simulink model "dummy"  (R2024b)
settings: Solver=VariableStepAuto  StartTime=0.0  StopTime=total_time  MaxStep=0.001  RelTol=1e-3
values from neighbouring files (symbols this model uses):
  D = diag([0.001, 0.001, 0.0175/6, 0.0175/6, 0.0175/6, 0.0175/6*Ts, 0.0175/6*Ts].^2)    [EX_opt_2.m]
  d = d_nom    (= 0.165)    [EX_opt_2.m]
  omega_wheels = sim_Tc_18.measures.signals.values(:,4:5)    [EX_opt_2.m]
  P_INIT_EKF = diag([0.001, 0.001, 0.0175/6, 0.0175/6, 0.0175/6, 0.0175/6*Ts, 0.0175/6*Ts].^2)    [EX_opt_2.m]
  PHI_INIT = [0; 0]    [EX_opt_2.m]
  prob_gps_loss = 0    [EX_opt_2.m]
  q = sim_Tc_18.measures.signals.values(:,1:3)    [EX_opt_2.m]
  Q_INIT_LOC = Q_INIT    [EX_opt_2.m]
  r = r_nom    (= 0.03)    [EX_opt_2.m]
  R_2 = diag([ENCODER_QUANTIZATION/6,ENCODER_QUANTIZATION/6].^2)    [EX_opt_2.m]
  R_5 = diag(([0.001, 0.001, 0.001, ENCODER_QUANTIZATION/6,ENCODER_QUANTIZATION/6]).^2)    [EX_opt_2.m]
  T_s = 0.04    [EX_opt_2.m]
  Ta = 1    [EX_opt_2.m]
  Tc = 18    [EX_opt_2.m]
  Ts = 0.04    [EX_opt_2.m]
  Z_INIT_EKF = [0; 0; 0; 0; 0; 0; 0]    [EX_opt_2.m]
undefined symbols (not defined in the file or in its folder): t_law
settings Model: Creator=alberto  LastModifiedBy=Enrico
settings DataIOCC: ReturnWorkspaceOutputs=off
settings RTWCC: GPUComputeCapability=3.5

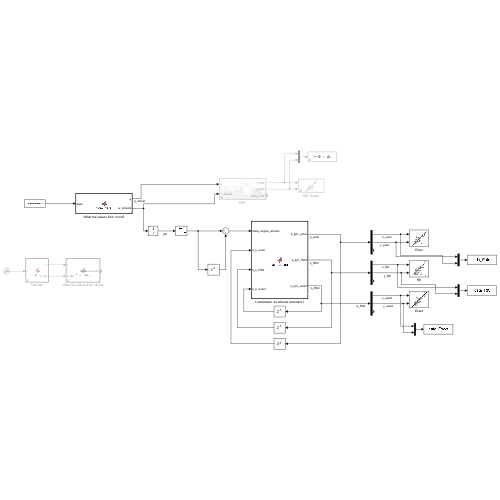
[thumbnail: Simulink's stored preview of the top-level diagram]
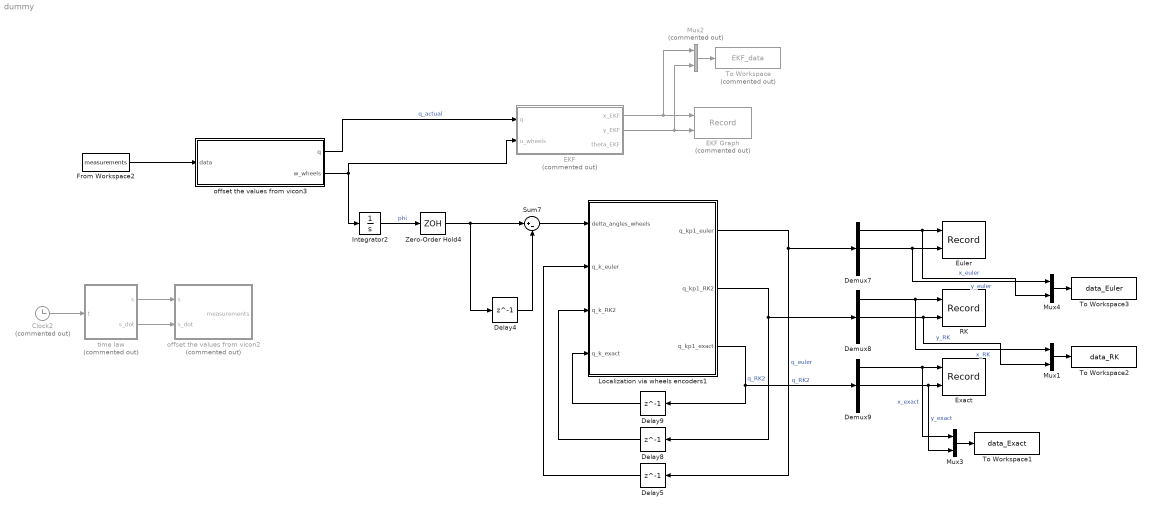
== system dummy ==
  Clock2 : Clock  Commented=on
      settings: Decimation=1/T_s
  Delay4 : Delay  DelayLength=1  InitialCondition=[0;0]  SampleTime=T_s
  Delay5 : Delay  DelayLength=1  InitialCondition=Q_INIT_LOC
  Delay8 : Delay  DelayLength=1  InitialCondition=Q_INIT_LOC
  Delay9 : Delay  DelayLength=1  InitialCondition=Q_INIT_LOC
  Demux7 : Demux  Outputs=3
  Demux8 : Demux  Outputs=3
  Demux9 : Demux  Outputs=3
  EKF : Subsystem  Commented=on
  EKF Graph : Record  Commented=on  FileSettingsInternal="{\"entries\":[{\"content\":{\"excelSettings\":{\"content\":{},\"type\":\"Streamout.ExcelSettings\"}},\"type\":\"Streamout.FileSettingStorage\",\"uuid\":\"\"}],\"packageUris\":[\"http:\\/\\/schema.mathworks.com\\/mf0\\/streamout_blocks\\/R2020a\"],\"version\":\"1.0\"}"  Layout=[1 1]  SignalsInternal="{\"entries\":[{\"content\":{},\"type\":\"RecordBlkView.InputSignals\",\"uuid\":\"\"}],\"packageUris\":[\"http:\\/\\/schema.mathworks.com\\/mf0\\/streamout_blocks\\/R2020a\"],\"version\":\"1.0\"}"  VisualizationBindings="{\"xyplotplugin\":{\"info\":[{\"series\":[],\"subplotID\":1}]}}"  CompatibilityTag=XY
  Euler : Record  FileSettingsInternal="{\"entries\":[{\"content\":{\"excelSettings\":{\"content\":{},\"type\":\"Streamout.ExcelSettings\"}},\"type\":\"Streamout.FileSettingStorage\",\"uuid\":\"\"}],\"packageUris\":[\"http:\\/\\/schema.mathworks.com\\/mf0\\/streamout_blocks\\/R2020a\"],\"version\":\"1.0\"}"  Layout=[1 1]  SignalsInternal="{\"entries\":[{\"content\":{\"signals\":[{\"content\":{\"blockPath\":[],\"dimensions\":[1,1],\"domain\":\"\",\"lineColor\":\"#edb120\",\"lineWidth\":2,\"plots\":[ 1 ],\"port\":1,\"sid\":[\"\"],\"signalID\":1,\"signalName\":\"x_euler\"},\"type\":\"RecordBlkView.Signal\",\"uuid\":\"\"},{\"content\":{\"blockPath\":[],\"dimensions\":[1,1],\"domain\":\"\",\"lineColor\":\"#b746ff\",\"lineWidth\":2,\"plots\":[ 1 ],\"port\":2,\"sid\":[\"\"],\"signalID\":2,\"signalName\":\"y_euler\"},\"type\":\"RecordBlkView.Signal\",\"uuid\":\"\"}]},\"type\":\"RecordBlkView.InputSignals\",\"uuid\":\"\"}],\"packageUris\":[\"http:\\/\\/schema.mathworks.com\\/mf0\\/streamout_blocks\\/R2020a\"],\"version\":\"1.0\"}"  VisualizationBindings="{\"xyplotplugin\":{\"info\":[{\"series\":[{\"bindingParametersList\":[{\"parameter\":\"X-Axis\",\"signalID\":1,\"signalName\":\"x_euler\"},{\"parameter\":\"Y-Axis\",\"signalID\":2,\"signalName\":\"y_euler\"}],\"seriesID\":0}],\"subplotID\":1}]}}"  CompatibilityTag=XY
  Exact : Record  FileSettingsInternal="{\"entries\":[{\"content\":{\"excelSettings\":{\"content\":{},\"type\":\"Streamout.ExcelSettings\"}},\"type\":\"Streamout.FileSettingStorage\",\"uuid\":\"\"}],\"packageUris\":[\"http:\\/\\/schema.mathworks.com\\/mf0\\/streamout_blocks\\/R2020a\"],\"version\":\"1.0\"}"  Layout=[1 1]  SignalsInternal="{\"entries\":[{\"content\":{\"signals\":[{\"content\":{\"blockPath\":[],\"dimensions\":[1,1],\"domain\":\"\",\"lineColor\":\"#ff6929\",\"lineWidth\":2,\"plots\":[ 1 ],\"port\":1,\"sid\":[\"\"],\"signalID\":1,\"signalName\":\"x_exact\"},\"type\":\"RecordBlkView.Signal\",\"uuid\":\"\"},{\"content\":{\"blockPath\":[],\"dimensions\":[1,1],\"domain\":\"\",\"lineColor\":\"#b746ff\",\"lineWidth\":2,\"plots\":[ 1 ],\"port\":2,\"sid\":[\"\"],\"signalID\":2,\"signalName\":\"y_exact\"},\"type\":\"RecordBlkView.Signal\",\"uuid\":\"\"}]},\"type\":\"RecordBlkView.InputSignals\",\"uuid\":\"\"}],\"packageUris\":[\"http:\\/\\/schema.mathworks.com\\/mf0\\/streamout_blocks\\/R2020a\"],\"version\":\"1.0\"}"  VisualizationBindings="{\"xyplotplugin\":{\"info\":[{\"series\":[{\"bindingParametersList\":[{\"parameter\":\"X-Axis\",\"signalID\":1,\"signalName\":\"x_exact\"},{\"parameter\":\"Y-Axis\",\"signalID\":2,\"signalName\":\"y_exact\"}],\"seriesID\":0}],\"subplotID\":1}]}}"  CompatibilityTag=XY
  From Workspace2 : FromWorkspace  VariableName=measurements  SampleTime=-1
  Integrator2 : Integrator  InitialCondition=PHI_INIT
  Localization via wheels encoders1 : MATLAB Function  TreatAsAtomicUnit=on
  Mux1 : Mux  Inputs=2
  Mux2 : Mux  Commented=on  Inputs=2
  Mux3 : Mux  Inputs=2
  Mux4 : Mux  Inputs=2
  RK : Record  FileSettingsInternal="{\"entries\":[{\"content\":{\"excelSettings\":{\"content\":{},\"type\":\"Streamout.ExcelSettings\"}},\"type\":\"Streamout.FileSettingStorage\",\"uuid\":\"\"}],\"packageUris\":[\"http:\\/\\/schema.mathworks.com\\/mf0\\/streamout_blocks\\/R2020a\"],\"version\":\"1.0\"}"  Layout=[1 1]  SignalsInternal="{\"entries\":[{\"content\":{\"signals\":[{\"content\":{\"blockPath\":[],\"dimensions\":[1,1],\"domain\":\"\",\"lineColor\":\"#ff6929\",\"lineWidth\":2,\"plots\":[ 1 ],\"port\":1,\"sid\":[\"\"],\"signalID\":1,\"signalName\":\"x_RK\"},\"type\":\"RecordBlkView.Signal\",\"uuid\":\"\"},{\"content\":{\"blockPath\":[],\"dimensions\":[1,1],\"domain\":\"\",\"lineColor\":\"#b746ff\",\"lineWidth\":2,\"plots\":[ 1 ],\"port\":2,\"sid\":[\"\"],\"signalID\":2,\"signalName\":\"y_RK\"},\"type\":\"RecordBlkView.Signal\",\"uuid\":\"\"}]},\"type\":\"RecordBlkView.InputSignals\",\"uuid\":\"\"}],\"packageUris\":[\"http:\\/\\/schema.mathworks.com\\/mf0\\/streamout_blocks\\/R2020a\"],\"version\":\"1.0\"}"  VisualizationBindings="{\"xyplotplugin\":{\"info\":[{\"series\":[{\"bindingParametersList\":[{\"parameter\":\"X-Axis\",\"signalID\":1,\"signalName\":\"x_RK\"},{\"parameter\":\"Y-Axis\",\"signalID\":2,\"signalName\":\"y_RK\"}],\"seriesID\":0}],\"subplotID\":1}]}}"  CompatibilityTag=XY
  Sum7 : Sum  Inputs=|+-
  To Workspace : ToWorkspace  Commented=on  VariableName=EKF_data  SampleTime=Ts
  To Workspace1 : ToWorkspace  VariableName=data_Exact  SampleTime=Ts
  To Workspace2 : ToWorkspace  VariableName=data_RK  SampleTime=Ts
  To Workspace3 : ToWorkspace  VariableName=data_Euler  SampleTime=Ts
  Zero-Order Hold4 : ZeroOrderHold  SampleTime=T_s
  offset the values from vicon2 : MATLAB Function  Commented=on  TreatAsAtomicUnit=on
  offset the values from vicon3 : MATLAB Function  TreatAsAtomicUnit=on
  time law : MATLAB Function  Commented=on  TreatAsAtomicUnit=on
  wires:
  EKF/2(y_EKF) -> Mux2/2, EKF Graph/2
  EKF/1(x_EKF) -> Mux2/1, EKF Graph/1
  Demux9/2 -> Mux3/2, Exact/2  "y_exact"
  Demux8/1 -> RK/1, Mux1/1  "x_RK"
  Demux8/2 -> Mux1/2, RK/2  "y_RK"
  Demux7/1 -> Mux4/2, Euler/1  "x_euler"
  Demux9/1 -> Mux3/1, Exact/1  "x_exact"
  Demux7/2 -> Mux4/1, Euler/2  "y_euler"
  Mux2/1 -> To Workspace/1
  Mux3/1 -> To Workspace1/1
  From Workspace2/1 -> offset the values from vicon3/1(data)
  Clock2/1 -> time law/1(t)
  time law/1(s) -> offset the values from vicon2/1(s)
  time law/2(s_dot) -> offset the values from vicon2/2(s_dot)
  offset the values from vicon3/1(q) -> EKF/1(q)  "q_actual"
  Delay5/1 -> Localization via wheels encoders1/2(q_k_euler)
  Localization via wheels encoders1/3(q_kp1_exact) -> Delay9/1, Demux9/1  "q_RK2"
  Localization via wheels encoders1/1(q_kp1_euler) -> Delay5/1, Demux7/1  "q_euler"
  offset the values from vicon3/2(w_wheels) -> Integrator2/1, EKF/2(u_wheels)
  Sum7/1 -> Localization via wheels encoders1/1(delta_angles_wheels)
  Delay8/1 -> Localization via wheels encoders1/3(q_k_RK2)
  Delay9/1 -> Localization via wheels encoders1/4(q_k_exact)
  Integrator2/1 -> Zero-Order Hold4/1  "phi"
  Localization via wheels encoders1/2(q_kp1_RK2) -> Delay8/1, Demux8/1  "q_RK2"
  Zero-Order Hold4/1 -> Sum7/1, Delay4/1
  Delay4/1 -> Sum7/2
  Mux1/1 -> To Workspace2/1
  Mux4/1 -> To Workspace3/1

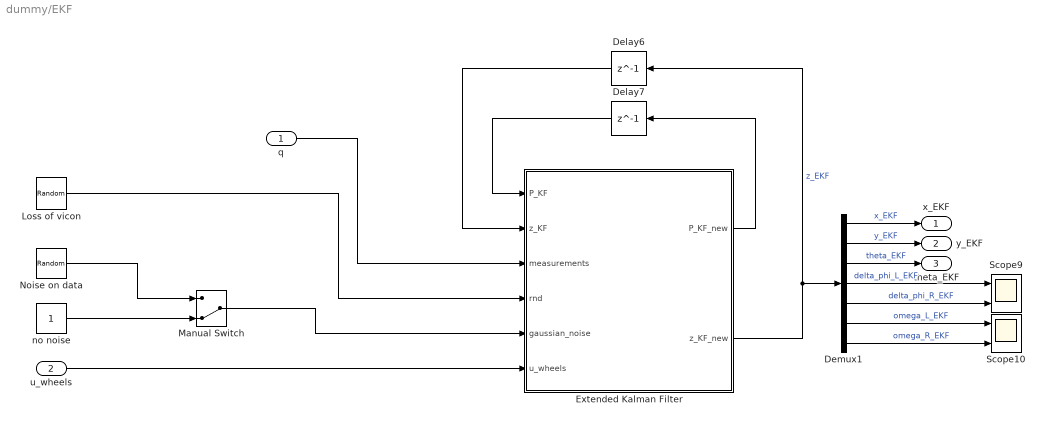
== system dummy/EKF ==
  q : Inport
  u_wheels : Inport  Port=2
  " Loss of vicon" : UniformRandomNumber  Minimum=0
  Delay6 : Delay  DelayLength=1  InitialCondition=Z_INIT_EKF
  Delay7 : Delay  DelayLength=1  InitialCondition=P_INIT_EKF
  Demux1 : Demux  Outputs=7
  Extended Kalman Filter : MATLAB Function  TreatAsAtomicUnit=on
  Manual Switch : ManualSwitch  CurrentSetting=0
  Noise on data : RandomNumber  Variance=0.0001
  Scope10 : Scope  NumInputPorts=2
  Scope9 : Scope  NumInputPorts=2
  no noise : Constant
  x_EKF : Outport
  y_EKF : Outport  Port=2
  theta_EKF : Outport  Port=3
  wires:
  Demux1/6 -> Scope10/1  "omega_L_EKF"
  Demux1/3 -> theta_EKF/1  "theta_EKF"
  Delay6/1 -> Extended Kalman Filter/2(z_KF)
  Delay7/1 -> Extended Kalman Filter/1(P_KF)
  Noise on data/1 -> Manual Switch/1
  Demux1/5 -> Scope9/2  "delta_phi_R_EKF"
  Demux1/7 -> Scope10/2  "omega_R_EKF"
  Extended Kalman Filter/1(P_KF_new) -> Delay7/1
  Manual Switch/1 -> Extended Kalman Filter/5(gaussian_noise)
  " Loss of vicon"/1 -> Extended Kalman Filter/4(rnd)
  Demux1/1 -> x_EKF/1  "x_EKF"
  Demux1/4 -> Scope9/1  "delta_phi_L_EKF"
  no noise/1 -> Manual Switch/2
  u_wheels/1 -> Extended Kalman Filter/6(u_wheels)
  Extended Kalman Filter/2(z_KF_new) -> Demux1/1, Delay6/1  "z_EKF"
  q/1 -> Extended Kalman Filter/3(measurements)
  Demux1/2 -> y_EKF/1  "y_EKF"

== matlab function dummy/offset the values from vicon2 ==
  data: s input; measurements output; s_dot input; q parameter; omega_wheels parameter
function measurements  = from_data(s, s_dot,q, omega_wheels)
    measurements = omega_wheels;
end

== matlab function dummy/offset the values from vicon3 ==
  data: data input; q output; w_wheels output
% function [q, w_wheels]  = from_data(data)
%     q = 0;
%     w_wheels = 0;
%     q(1) = data(1);
%     q(2) = data(2);
%     q(3) = data(3);
%     w_wheels(1) = data(4);
%     w_wheels(2) = data(5);
% 
% end
function [q, w_wheels] = from_data(data)
    q = data(1:3);         % [x; y; theta]
    w_wheels = data(4:5);  % [omega_R; omega_L]
end

== matlab function dummy/EKF/Extended Kalman Filter ==
  data: P_KF input; P_KF_new output; z_KF input; measurements input; D parameter; R_2 parameter; R_5 parameter; T_s parameter; r parameter; d parameter; prob_gps_loss parameter; rnd input; gaussian_noise input; z_KF_new output; u_wheels input
function [P_KF_new, z_KF_new] = EKF_filtering(P_KF, z_KF, measurements, D, R_2, R_5 ,T_s, r, d, prob_gps_loss, rnd, gaussian_noise,u_wheels)

% z_KF = [x_EKF, y_EKF, theta_EKF, delta_phi_L_EKF, delta_phi_R_EKF, omega_L_EKF, omega_R_EKF]

v_k = r * (z_KF(6) + z_KF(7))/2;
w_k = r * (z_KF(7) - z_KF(6))/d;

theta_mean = z_KF(3) + (w_k * T_s)/2;

F_k = [1, 0, -T_s * v_k * sin(theta_mean), 0, 0, T_s * r * cos(theta_mean)/2 + (T_s)^2 * r * v_k * sin(theta_mean)/(2*d), T_s * r * cos(theta_mean)/2 - (T_s)^2 * r * v_k * sin(theta_mean)/(2*d);
       0, 1,  T_s * v_k * cos(theta_mean), 0, 0, T_s * r * sin(theta_mean)/2 + (T_s)^2 * r * v_k * cos(theta_mean)/(2*d), T_s * r * sin(theta_mean)/2 - (T_s)^2 * r * v_k * cos(theta_mean)/(2*d);
       0, 0, 1, 0, 0, (-T_s*r)/d, (T_s*r)/d;
       0, 0, 0, 0, 0, T_s, 0;
       0, 0, 0, 0, 0, 0, T_s;
       0, 0, 0, 0, 0, 0, 0;
       0, 0, 0, 0, 0, 0, 0];

%% Prediction part

z_pred = [z_KF(1)+(T_s*r*(z_KF(6)+z_KF(7))/2)*cos(theta_mean + (T_s*r*(z_KF(6)+z_KF(7)))/(2*d));
          z_KF(2)+(T_s*r*(z_KF(6)+z_KF(7))/2)*sin(theta_mean + (T_s*r*(z_KF(7)-z_KF(6)))/(2*d));
          theta_mean + (T_s*r*(z_KF(7)-z_KF(6))/(2*d));
          T_s*z_KF(6);
          T_s*z_KF(7);
          u_wheels(1);
          u_wheels(2)];

P_pred = F_k * P_KF * F_k' + D;


%% Update

if(rnd<prob_gps_loss)

    % Just encoders
    y_measurement = [measurements(4); measurements(5)];
    H = [0, 0, 0, 0, 0, 1, 0;
         0, 0, 0, 0, 0, 0, 1];

    e = y_measurement - H * z_pred;
    K = P_pred * H' /(H * P_pred * H' + R_2);

    z_KF_new = z_pred +  K * e;
    P_KF_new = P_pred - K * H * P_pred;

else 
    % GPS(x,y,yaw) + Encoders(omegaL,omegaR)
    y_measurement = [measurements(1)+gaussian_noise;measurements(2)+gaussian_noise;measurements(3)+gaussian_noise; measurements(4); measurements(5)];
    
    H = [1, 0, 0, 0, 0, 0, 0;
         0, 1, 0, 0, 0, 0, 0;
         0, 0, 1, 0, 0, 0, 0;
         0, 0, 0, 0, 0, 1, 0;
         0, 0, 0, 0, 0, 0, 1];

    e = y_measurement - H * z_pred;
    K = P_pred * H' /(H * P_pred * H' + R_5);

    z_KF_new = z_pred + K * e;
    P_KF_new = P_pred - K * H * P_pred;
end

== matlab function dummy/Localization via wheels encoders1 ==
  data: delta_angles_wheels input; q_k_euler input; q_k_RK2 input; q_k_exact input; r parameter; d parameter; q_kp1_euler output; T_s parameter; q_kp1_RK2 output; q_kp1_exact output
function [q_kp1_euler, q_kp1_RK2, q_kp1_exact] = localization(delta_angles_wheels, q_k_euler, q_k_RK2, q_k_exact, r, d, T_s)

    v_k = r * (delta_angles_wheels(1) + delta_angles_wheels(2)) / (T_s * 2);
    w_k = r * (delta_angles_wheels(2) - delta_angles_wheels(1)) / (T_s * d);
    
    % Euler integration
    x_kp1_euler     = q_k_euler(1) + T_s * v_k * cos(q_k_euler(3));
    y_kp1_euler     = q_k_euler(2) + T_s * v_k * sin(q_k_euler(3));
    theta_kp1_euler = q_k_euler(3) + T_s * w_k;
    q_kp1_euler     = [x_kp1_euler; y_kp1_euler; theta_kp1_euler];
    
    % Runge-Kutta 2
    x_kp1_RK2       = q_k_RK2(1) + T_s * v_k * cos(q_k_RK2(3) + T_s * w_k / 2);
    y_kp1_RK2       = q_k_RK2(2) + T_s * v_k * sin(q_k_RK2(3) + T_s * w_k / 2);
    theta_kp1_RK2   = q_k_RK2(3) + T_s * w_k;
    q_kp1_RK2       = [x_kp1_RK2; y_kp1_RK2; theta_kp1_RK2];
    
    % Exact Integration
    x_kp1_exact     = q_k_exact(1) + (v_k / w_k) * (sin(q_k_exact(3) + w_k*T_s) - sin(q_k_exact(3)));
    y_kp1_exact     = q_k_exact(2) - (v_k / w_k) * (cos(q_k_exact(3) + w_k*T_s) - cos(q_k_exact(3)));
    theta_kp1_exact = q_k_exact(3) + T_s * w_k;
    
    % The problem with Exact integration fixed by switching strategy
    if abs(delta_angles_wheels(2) - delta_angles_wheels(1)) <= 0.001
        q_kp1_exact = [x_kp1_RK2; y_kp1_RK2; theta_kp1_RK2];
    else
        q_kp1_exact = [x_kp1_exact; y_kp1_exact; theta_kp1_exact];
    end

end

== matlab function dummy/time law ==
  data: s output; t input; Ta parameter; s_dot output; Tc parameter; t_law parameter
function [s,s_dot]=fcn(t, Ta, Tc, t_law)

    v_c = 1 / (Ta + Tc);
    a = v_c / Ta;

    if (t_law == 0)
        s_dot = 1/Tc;
        s = s_dot * t;

        if(t > Tc)
            s_dot = 0;
            s = 1;
        end
    else
        if(t > 2*Ta+Tc)
            s_dot = 0;
            s = 1;
        elseif(t > Ta+Tc)
            s_dot = v_c - a * (t - Ta - Tc);
            s = (a * Ta^2)/2 + v_c * (Tc) + (a * (t - Tc - Ta)^2)/2;
        elseif(t > Ta)
            s_dot = v_c; 
            s = (a * Ta^2)/2 + v_c * (t - Ta);
        else 
            s_dot = a * t;
            s = (a * t^2)/2;
        end
    end
end
